simulink model "Pendulo"  (R2015a)
settings: Solver=ode45  StartTime=0.0  StopTime=10.0  RelTol=1e-3
undefined symbols (not defined in the file): B, g, J, l, m
settings Model: Creator=Henry Alberto  LastModifiedBy=Henry Alberto

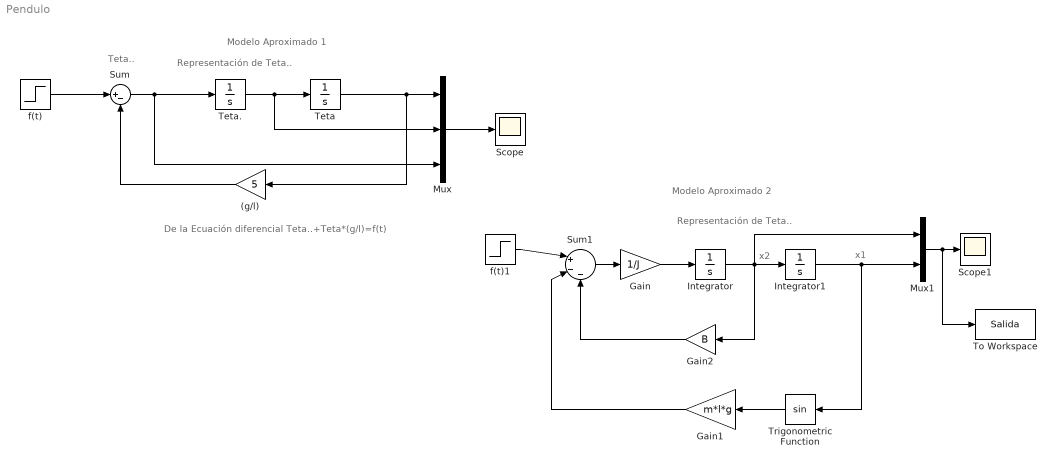
== system Pendulo ==
  note: x1
  note: x2
  note: Teta..
  note: Modelo Aproximado 1
  note: De la Ecuación diferencial Teta..+Teta*(g/l)=f(t)
  note: Representación de Teta..
  note: Modelo Aproximado 2
  note: Representación de Teta..
  (g/l) : Gain  Gain=5
  Gain : Gain  Gain=1/J
  Gain1 : Gain  Gain=m*l*g
  Gain2 : Gain  Gain=B
  Integrator : Integrator
  Integrator1 : Integrator
  Mux : Mux  Inputs=3
  Mux1 : Mux  Inputs=2
  Scope : Scope
      settings: ShowLegends=on
  Scope1 : Scope
  Sum : Sum  Inputs=|+-
  Sum1 : Sum  Inputs=|+--
  Teta : Integrator  InitialCondition=pi/2
  Teta. : Integrator  InitialCondition=2*pi
  To Workspace : ToWorkspace  VariableName=Salida  SaveFormat=Timeseries  SampleTime=-1
  Trigonometric Function : Trigonometry
  f(t) : Step  Time=2  SampleTime=0
  f(t)1 : Step  Time=2  SampleTime=0
  wires:
  Teta./1 -> Mux/2, Teta/1
  Sum/1 -> Mux/3, Teta./1
  Teta/1 -> (g/l)/1, Mux/1
  (g/l)/1 -> Sum/2
  f(t)/1 -> Sum/1
  Mux/1 -> Scope/1
  Sum1/1 -> Gain/1
  Gain/1 -> Integrator/1
  Integrator/1 -> Mux1/1, Gain2/1, Integrator1/1
  Integrator1/1 -> Trigonometric Function/1, Mux1/2
  Trigonometric Function/1 -> Gain1/1
  Gain2/1 -> Sum1/3
  Gain1/1 -> Sum1/2
  f(t)1/1 -> Sum1/1
  Mux1/1 -> To Workspace/1, Scope1/1
